simulink model "singletrack_model_ROS"  (R2018b)
settings: Solver=VariableStepAuto  StartTime=0.0  StopTime=20.0  RelTol=1e-3
values from neighbouring files (symbols this model uses):
  actuation_delay = 0.09    [init_singletrack.m]
  car_param = [a, b, Cf, Cr, Iz, m]    [init_singletrack.m]
  car_state0 = [psi0, r0, beta0, x0, y0]    [init_singletrack.m]
  meas_Ts = 0.001    [init_singletrack.m]
  ROS_clockPublishingPeriod = 1.0e-2    (= 0.01)    [initParameters.m]    (also in init_singletrack.m = 0.0005)
  ROS_statePublishingPeriod = 2.0e-2    (= 0.02)    [initParameters.m]    (also in init_singletrack.m = 0.01)
undefined symbols (not defined in the file or in its folder): Clock_, singleTrack_model, Theta, X, Y
libraries: robotlib x14
settings Model: Creator=bascetta  LastModifiedBy=bascetta
settings SFSimCC: SimUseLocalCustomCode=off
settings RTWCC: RTWUseLocalCustomCode=off

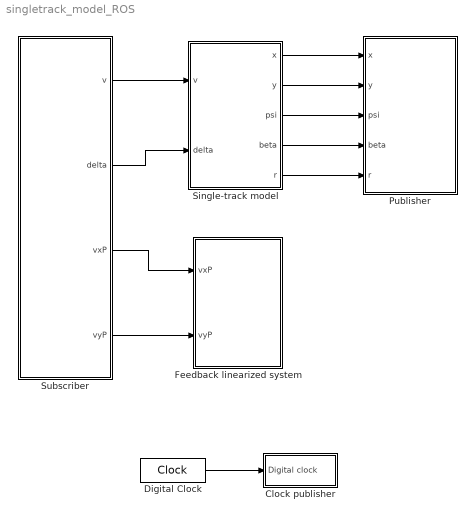
== system singletrack_model_ROS ==
  Clock publisher : Subsystem
  Digital Clock : DigitalClock  SampleTime=ROS_clockPublishingPeriod
  Feedback linearized system : Subsystem
  Publisher : Subsystem
  Single-track model : Subsystem  mask{car_parameters=car_param}
      mask prompts: car_parameters "Car parameters"
  Subscriber : Subsystem
  wires:
  Single-track model/3(psi) -> Publisher/3(psi)
  Single-track model/4(beta) -> Publisher/4(beta)
  Subscriber/1(v) -> Single-track model/1(v)
  Subscriber/2(delta) -> Single-track model/2(delta)
  Single-track model/5(r) -> Publisher/5(r)
  Single-track model/2(y) -> Publisher/2(y)
  Single-track model/1(x) -> Publisher/1(x)
  Digital Clock/1 -> Clock publisher/1(Digital clock)
  Subscriber/3(vxP) -> Feedback linearized system/1(vxP)
  Subscriber/4(vyP) -> Feedback linearized system/2(vyP)

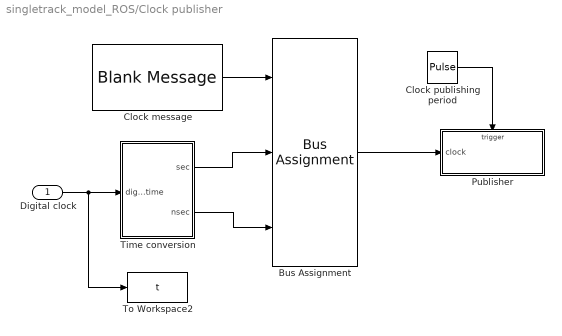
== system singletrack_model_ROS/Clock publisher ==
  Digital clock : Inport
  Bus Assignment : BusAssignment  DialogController=Simulink.DDGSource_BusAssignment  AssignedSignals=Clock_.Sec,Clock_.Nsec
  Clock message : robotlib/Blank Message  messageType=rosgraph_msgs/Clock  SampleTime=inf
      settings: SourceProductBaseCode=RO
  Clock publishing period : DiscretePulseGenerator  PulseType=Time based  Period=ROS_clockPublishingPeriod  PulseWidth=50
  Publisher : Subsystem  TreatAsAtomicUnit=on
  Time conversion : MATLAB Function  TreatAsAtomicUnit=on
  To Workspace2 : ToWorkspace  VariableName=t  SampleTime=meas_Ts
      settings: Save2DSignal=2-D array (concatenate along first dimension)
  wires:
  Clock message/1 -> Bus Assignment/1
  Bus Assignment/1 -> Publisher/1(clock)
  Time conversion/1(sec) -> Bus Assignment/2
  Time conversion/2(nsec) -> Bus Assignment/3
  Digital clock/1 -> To Workspace2/1, Time conversion/1(digital_time)
  Clock publishing period/1 -> Publisher/Trigger

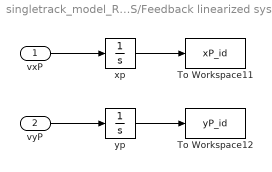
== system singletrack_model_ROS/Feedback linearized system ==
  vxP : Inport
  vyP : Inport  Port=2
  " xp " : Integrator  InitialCondition=car_state0(4)
  " yp " : Integrator  InitialCondition=car_state0(5)
  To Workspace11 : ToWorkspace  VariableName=xP_id  SampleTime=meas_Ts
      settings: Save2DSignal=2-D array (concatenate along first dimension)
  To Workspace12 : ToWorkspace  VariableName=yP_id  SampleTime=meas_Ts
      settings: Save2DSignal=2-D array (concatenate along first dimension)
  wires:
  vyP/1 -> " yp "/1
  vxP/1 -> " xp "/1
  " yp "/1 -> To Workspace12/1
  " xp "/1 -> To Workspace11/1

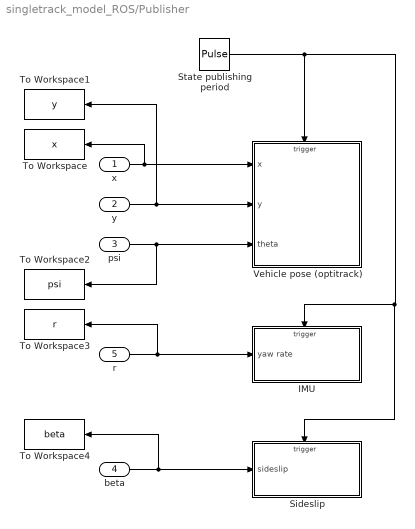
== system singletrack_model_ROS/Publisher ==
  x : Inport
  y : Inport  Port=2
  psi : Inport  Port=3
  beta : Inport  Port=4
  r : Inport  Port=5
  IMU : Subsystem  TreatAsAtomicUnit=on
  Sideslip : Subsystem  TreatAsAtomicUnit=on
  State publishing period : DiscretePulseGenerator  PulseType=Time based  Period=ROS_statePublishingPeriod  PulseWidth=50
  To Workspace : ToWorkspace  VariableName=x  SampleTime=meas_Ts
      settings: Save2DSignal=2-D array (concatenate along first dimension)
  To Workspace1 : ToWorkspace  VariableName=y  SampleTime=meas_Ts
      settings: Save2DSignal=2-D array (concatenate along first dimension)
  To Workspace2 : ToWorkspace  VariableName=psi  SampleTime=meas_Ts
      settings: Save2DSignal=2-D array (concatenate along first dimension)
  To Workspace3 : ToWorkspace  VariableName=r  SampleTime=meas_Ts
      settings: Save2DSignal=2-D array (concatenate along first dimension)
  To Workspace4 : ToWorkspace  VariableName=beta  SampleTime=meas_Ts
      settings: Save2DSignal=2-D array (concatenate along first dimension)
  Vehicle pose (optitrack) : Subsystem  TreatAsAtomicUnit=on
  wires:
  State publishing period/1 -> Sideslip/Trigger, IMU/Trigger, Vehicle pose (optitrack)/Trigger
  x/1 -> To Workspace/1, Vehicle pose (optitrack)/1(x)
  y/1 -> To Workspace1/1, Vehicle pose (optitrack)/2(y)
  psi/1 -> To Workspace2/1, Vehicle pose (optitrack)/3(theta)
  r/1 -> To Workspace3/1, IMU/1(yaw rate)
  beta/1 -> To Workspace4/1, Sideslip/1(sideslip)

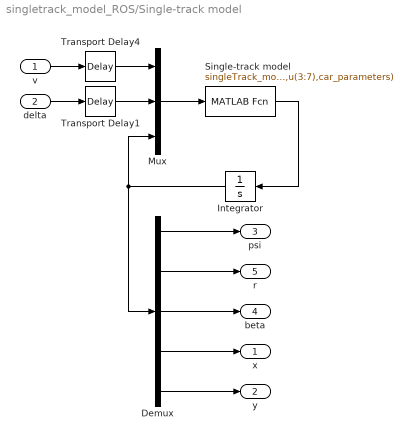
== system singletrack_model_ROS/Single-track model ==
  v : Inport
  delta : Inport  Port=2
  Demux : Demux  Outputs=5
  Integrator : Integrator  InitialCondition=car_state0
  Mux : Mux  Inputs=3
  Single-track model : MATLABFcn  MATLABFcn=singleTrack_model(u(1:2),u(3:7),car_parameters)  OutputDimensions=5
  Transport Delay1 : TransportDelay  DelayTime=actuation_delay
  Transport Delay4 : TransportDelay  DelayTime=actuation_delay
  x : Outport
  y : Outport  Port=2
  psi : Outport  Port=3
  beta : Outport  Port=4
  r : Outport  Port=5
  wires:
  Integrator/1 -> Demux/1, Mux/3
  Single-track model/1 -> Integrator/1
  delta/1 -> Transport Delay1/1
  Demux/4 -> x/1
  Mux/1 -> Single-track model/1
  Demux/5 -> y/1
  Demux/3 -> beta/1
  v/1 -> Transport Delay4/1
  Demux/2 -> r/1
  Demux/1 -> psi/1
  Transport Delay4/1 -> Mux/1
  Transport Delay1/1 -> Mux/2

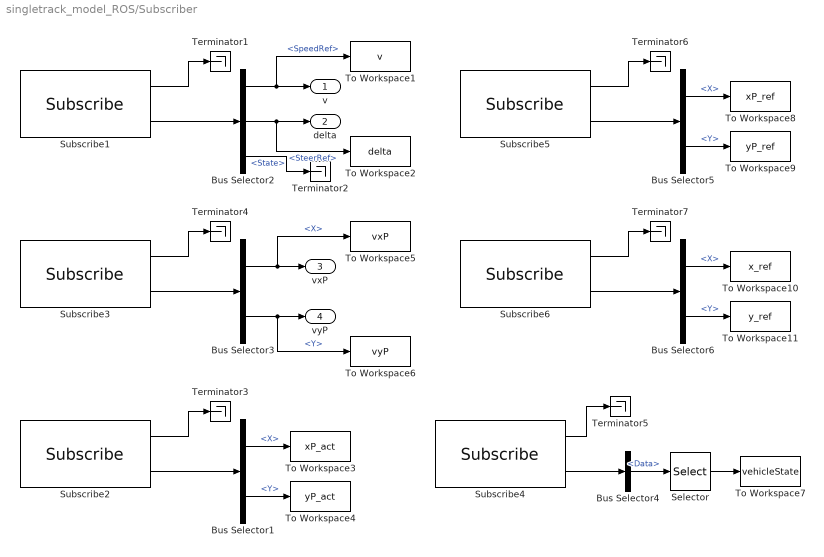
== system singletrack_model_ROS/Subscriber ==
  Bus Selector1 : BusSelector  OutputSignals=Point.X,Point.Y
  Bus Selector2 : BusSelector  OutputSignals=SpeedRef,SteerRef,State
  Bus Selector3 : BusSelector  OutputSignals=Twist.Linear.X,Twist.Linear.Y
  Bus Selector4 : BusSelector  OutputSignals=Data
  Bus Selector5 : BusSelector  OutputSignals=Point.X,Point.Y
  Bus Selector6 : BusSelector  OutputSignals=Point.X,Point.Y
  Selector : Selector  InputPortWidth=128  IndexOptions=Starting index (dialog)  Indices=1  OutputSizes=9
  Subscribe1 : robotlib/Subscribe  topicSource=Specify your own  topic=/controller_cmd  messageType=car_msgs/car_cmd  sampleTime=-1  messageQueueLength=1
      settings: SourceProductBaseCode=RO
  Subscribe2 : robotlib/Subscribe  topicSource=Specify your own  topic=/feedback_linearization/pointP_actPos  messageType=geometry_msgs/PointStamped  sampleTime=-1  messageQueueLength=1
      settings: SourceProductBaseCode=RO
  Subscribe3 : robotlib/Subscribe  topicSource=Specify your own  topic=/feedback_linearization/pointP_actVel  messageType=geometry_msgs/TwistStamped  sampleTime=-1  messageQueueLength=1
      settings: SourceProductBaseCode=RO
  Subscribe4 : robotlib/Subscribe  topicSource=Specify your own  topic=/feedback_linearization/vehicleState  messageType=std_msgs/Float64MultiArray  sampleTime=-1  messageQueueLength=1
      settings: SourceProductBaseCode=RO
  Subscribe5 : robotlib/Subscribe  topicSource=Specify your own  topic=/feedback_linearization/pointP_refPos  messageType=geometry_msgs/PointStamped  sampleTime=-1  messageQueueLength=1
      settings: SourceProductBaseCode=RO
  Subscribe6 : robotlib/Subscribe  topicSource=Specify your own  topic=/feedback_linearization/vehicle_refPos  messageType=geometry_msgs/PointStamped  sampleTime=-1  messageQueueLength=1
      settings: SourceProductBaseCode=RO
  Terminator{1..7} (7 alike) : Terminator
  To Workspace1 : ToWorkspace  VariableName=v  SampleTime=meas_Ts
      settings: Save2DSignal=2-D array (concatenate along first dimension)
  To Workspace10 : ToWorkspace  VariableName=x_ref  SampleTime=meas_Ts
      settings: Save2DSignal=2-D array (concatenate along first dimension)
  To Workspace11 : ToWorkspace  VariableName=y_ref  SampleTime=meas_Ts
      settings: Save2DSignal=2-D array (concatenate along first dimension)
  To Workspace2 : ToWorkspace  VariableName=delta  SampleTime=meas_Ts
      settings: Save2DSignal=2-D array (concatenate along first dimension)
  To Workspace3 : ToWorkspace  VariableName=xP_act  SampleTime=meas_Ts
      settings: Save2DSignal=2-D array (concatenate along first dimension)
  To Workspace4 : ToWorkspace  VariableName=yP_act  SampleTime=meas_Ts
      settings: Save2DSignal=2-D array (concatenate along first dimension)
  To Workspace5 : ToWorkspace  VariableName=vxP  SampleTime=meas_Ts
      settings: Save2DSignal=2-D array (concatenate along first dimension)
  To Workspace6 : ToWorkspace  VariableName=vyP  SampleTime=meas_Ts
      settings: Save2DSignal=2-D array (concatenate along first dimension)
  To Workspace7 : ToWorkspace  VariableName=vehicleState  SampleTime=meas_Ts
      settings: Save2DSignal=2-D array (concatenate along first dimension)
  To Workspace8 : ToWorkspace  VariableName=xP_ref  SampleTime=meas_Ts
      settings: Save2DSignal=2-D array (concatenate along first dimension)
  To Workspace9 : ToWorkspace  VariableName=yP_ref  SampleTime=meas_Ts
      settings: Save2DSignal=2-D array (concatenate along first dimension)
  v : Outport
  delta : Outport  Port=2
  vxP : Outport  Port=3
  vyP : Outport  Port=4
  wires:
  Subscribe1/1 -> Terminator1/1
  Subscribe1/2 -> Bus Selector2/1
  Bus Selector2/1 -> To Workspace1/1, v/1  "<SpeedRef>"
  Bus Selector2/2 -> To Workspace2/1, delta/1  "<SteerRef>"
  Bus Selector2/3 -> Terminator2/1  "<State>"
  Subscribe2/1 -> Terminator3/1
  Subscribe2/2 -> Bus Selector1/1
  Bus Selector1/1 -> To Workspace3/1  "<X>"
  Bus Selector1/2 -> To Workspace4/1  "<Y>"
  Bus Selector3/2 -> vyP/1, To Workspace6/1  "<Y>"
  Subscribe3/1 -> Terminator4/1
  Bus Selector3/1 -> vxP/1, To Workspace5/1  "<X>"
  Subscribe4/1 -> Terminator5/1
  Subscribe4/2 -> Bus Selector4/1
  Bus Selector4/1 -> Selector/1  "<Data>"
  Selector/1 -> To Workspace7/1
  Subscribe5/1 -> Terminator6/1
  Bus Selector5/1 -> To Workspace8/1  "<X>"
  Bus Selector5/2 -> To Workspace9/1  "<Y>"
  Subscribe5/2 -> Bus Selector5/1
  Subscribe3/2 -> Bus Selector3/1
  Subscribe6/1 -> Terminator7/1
  Bus Selector6/1 -> To Workspace10/1  "<X>"
  Bus Selector6/2 -> To Workspace11/1  "<Y>"
  Subscribe6/2 -> Bus Selector6/1

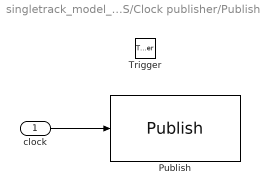
== system singletrack_model_ROS/Clock publisher/Publisher ==
  clock : Inport
  Trigger : TriggerPort  VariantControl=Variant
  Publish : robotlib/Publish  topicSource=Specify your own  topic=/clock  messageType=rosgraph_msgs/Clock  messageQueueLength=1
      settings: SourceProductBaseCode=RO
  wires:
  clock/1 -> Publish/1

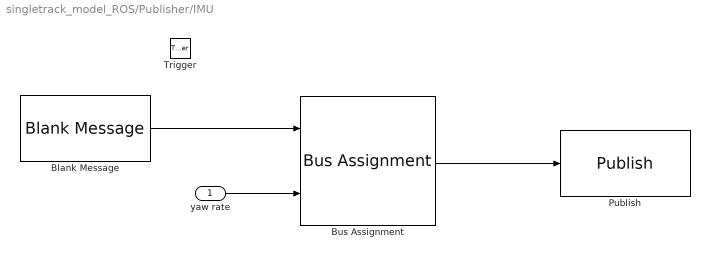
== system singletrack_model_ROS/Publisher/IMU ==
  yaw rate : Inport
  Trigger : TriggerPort  VariantControl=Variant
  Blank Message : robotlib/Blank Message  messageType=sensor_msgs/Imu  SampleTime=inf
      settings: SourceProductBaseCode=RO
  Bus Assignment : BusAssignment  DialogController=Simulink.DDGSource_BusAssignment  AssignedSignals=AngularVelocity.Z
  Publish : robotlib/Publish  topicSource=Specify your own  topic=/imu/data  messageType=sensor_msgs/Imu  messageQueueLength=1
      settings: SourceProductBaseCode=RO
  wires:
  Blank Message/1 -> Bus Assignment/1
  Bus Assignment/1 -> Publish/1
  yaw rate/1 -> Bus Assignment/2

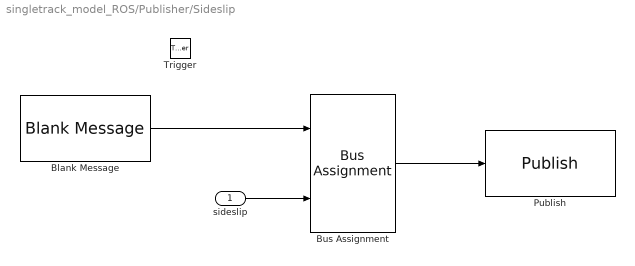
== system singletrack_model_ROS/Publisher/Sideslip ==
  sideslip : Inport
  Trigger : TriggerPort  VariantControl=Variant
  Blank Message : robotlib/Blank Message  messageType=std_msgs/Float64  SampleTime=inf
      settings: SourceProductBaseCode=RO
  Bus Assignment : BusAssignment  DialogController=Simulink.DDGSource_BusAssignment  AssignedSignals=Data
  Publish : robotlib/Publish  topicSource=Specify your own  topic=/car_simulator/sideslip  messageType=std_msgs/Float64  messageQueueLength=1
      settings: SourceProductBaseCode=RO
  wires:
  Blank Message/1 -> Bus Assignment/1
  Bus Assignment/1 -> Publish/1
  sideslip/1 -> Bus Assignment/2

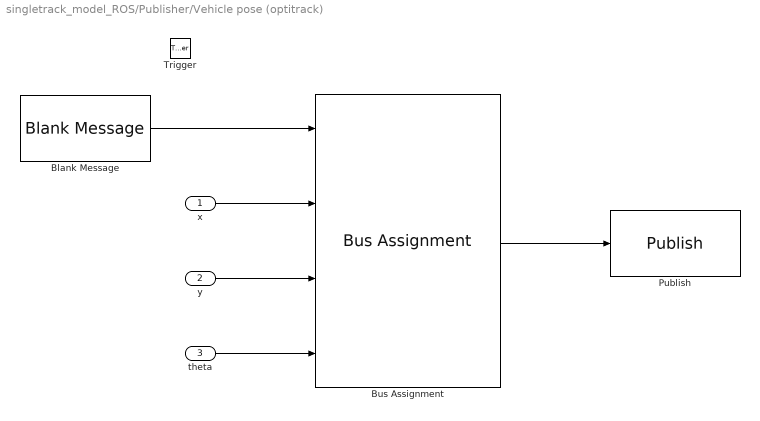
== system singletrack_model_ROS/Publisher/Vehicle pose (optitrack) ==
  x : Inport
  y : Inport  Port=2
  theta : Inport  Port=3
  Trigger : TriggerPort  VariantControl=Variant
  Blank Message : robotlib/Blank Message  messageType=geometry_msgs/Pose2D  SampleTime=inf
      settings: SourceProductBaseCode=RO
  Bus Assignment : BusAssignment  DialogController=Simulink.DDGSource_BusAssignment  AssignedSignals=X,Y,Theta
  Publish : robotlib/Publish  topicSource=Specify your own  topic=/car/ground_pose  messageType=geometry_msgs/Pose2D  messageQueueLength=1
      settings: SourceProductBaseCode=RO
  wires:
  Blank Message/1 -> Bus Assignment/1
  Bus Assignment/1 -> Publish/1
  x/1 -> Bus Assignment/2
  y/1 -> Bus Assignment/3
  theta/1 -> Bus Assignment/4

== matlab function singletrack_model_ROS/Clock publisher/Time conversion ==
  data: digital_time input; sec output; nsec output
function [sec,nsec] = time2rosclock(digital_time)

sec = floor(digital_time);
nsec = round((digital_time-sec)*1.0e+9);
